simulink model "exp5_1"  (Simulink 3.00)
settings: Solver=ode45  StartTime=0.0  StopTime=20  MaxStep=1e-3  RelTol=1e-3
libraries: simulink_extras x1

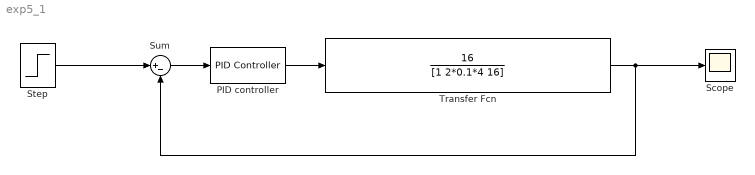
== system exp5_1 ==
  PID controller : simulink_extras/Additional Linear/PID Controller  P=5  I=10  D=1
  Scope : Scope
      settings: TimeRange=20  YMin=0  YMax=1.4  SaveToWorkspace=off  SaveName=ScopeData  LimitMaxRows=off
  Step : Step  Time=0  Before=0  After=1  SampleTime=0
  Sum : Sum  Inputs=|+-  SaturateOnIntegerOverflow=on
  Transfer Fcn : TransferFcn  Numerator=[16]  Denominator=[1 2*0.1*4 16]
  wires:
  Transfer Fcn/1 -> Scope/1, Sum/2
  Step/1 -> Sum/1
  Sum/1 -> PID controller/1
  PID controller/1 -> Transfer Fcn/1
